simulink model "traj_model_pid"  (R2022b)
settings: Solver=VariableStepAuto  StartTime=0.0  StopTime=10.0  RelTol=1e-3
values from neighbouring files (symbols this model uses):
  L = 235    [trajectory_script.m]
  v_d = 100    [trajectory_script.m]
settings Model: Creator=hamra  LastModifiedBy=hamra

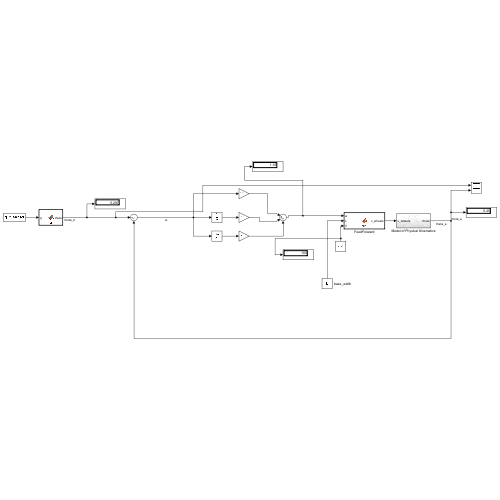
[thumbnail: Simulink's stored preview of the top-level diagram]
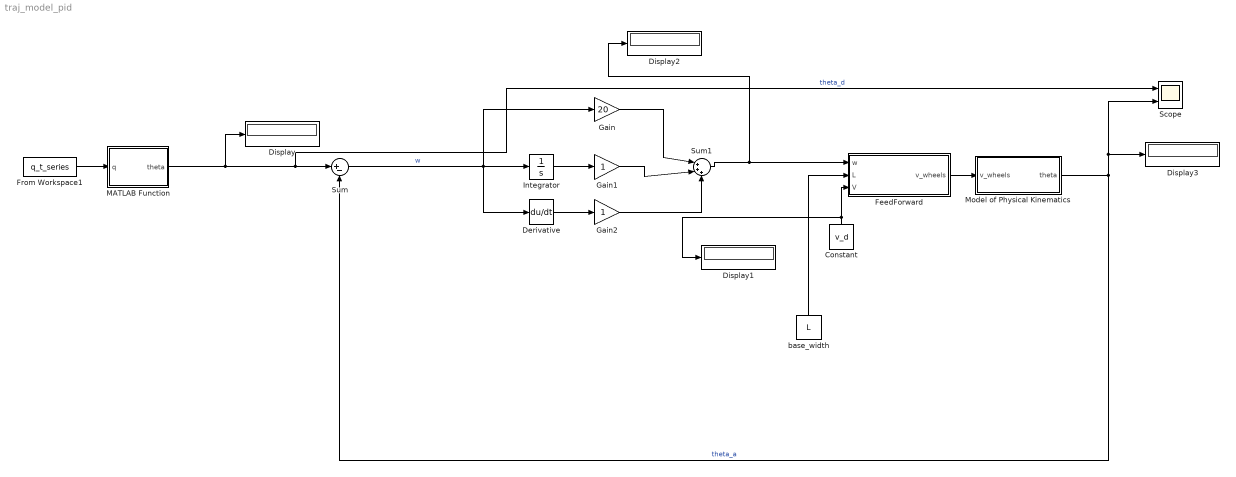
== system traj_model_pid ==
  Constant : Constant  Value=v_d
  Derivative : Derivative
  Display{,1..3} (4 alike) : Display
  FeedForward : MATLAB Function  TreatAsAtomicUnit=on
  From Workspace1 : FromWorkspace  VariableName=q_t_series
  Gain : Gain  Gain=20
  Gain1 : Gain
  Gain2 : Gain
  Integrator : Integrator
  MATLAB Function : MATLAB Function  TreatAsAtomicUnit=on
  Model of Physical Kinematics : Subsystem
  Scope : Scope  NumInputPorts=2
  Sum : Sum  Inputs=|+-
  Sum1 : Sum  Inputs=|+++
  base_width : Constant  Value=L
  wires:
  From Workspace1/1 -> MATLAB Function/1(q)
  Sum/1 -> Derivative/1, Gain/1, Integrator/1  "w"
  Derivative/1 -> Gain2/1
  Integrator/1 -> Gain1/1
  Gain/1 -> Sum1/1
  Gain1/1 -> Sum1/2
  Gain2/1 -> Sum1/3
  base_width/1 -> FeedForward/2(L)
  FeedForward/1(v_wheels) -> Model of Physical Kinematics/1(v_wheels)
  Constant/1 -> FeedForward/3(V), Display1/1
  Model of Physical Kinematics/1(theta) -> Scope/2, Display3/1, Sum/2  "theta_a"
  MATLAB Function/1(theta) -> Display/1, Scope/1, Sum/1  "theta_d"
  Sum1/1 -> Display2/1, FeedForward/1(w)

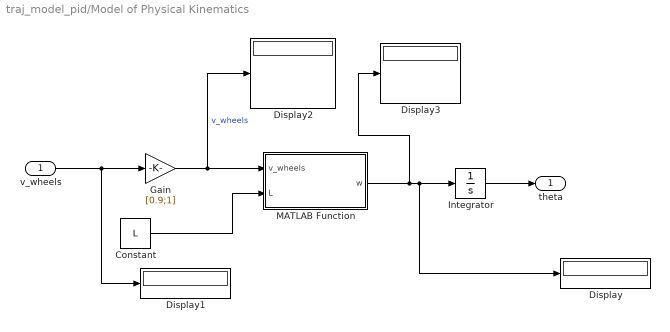
== system traj_model_pid/Model of Physical Kinematics ==
  v_wheels : Inport
  Constant : Constant  Value=L
  Display{,1..3} (4 alike) : Display
  Gain : Gain  Gain=[0.9;1]
  Integrator : Integrator
  MATLAB Function : MATLAB Function  TreatAsAtomicUnit=on
  theta : Outport
  wires:
  Constant/1 -> MATLAB Function/2(L)
  MATLAB Function/1(w) -> Display3/1, Display/1, Integrator/1
  Gain/1 -> Display2/1, MATLAB Function/1(v_wheels)  "v_wheels"
  Integrator/1 -> theta/1
  v_wheels/1 -> Display1/1, Gain/1

== matlab function traj_model_pid/MATLAB Function ==
  data: q input; theta output
function theta = fcn(q)

theta = q(3);

== matlab function traj_model_pid/Model of Physical Kinematics/MATLAB Function ==
  data: v_wheels input; w output; L input
function w = fcn(v_wheels, L)

v_r = v_wheels(1);
v_l = v_wheels(2);

w = (v_r - v_l)/L;

== matlab function traj_model_pid/FeedForward ==
  data: w input; v_wheels output; L input; V input
function v_wheels = fcn(w,L, V)
%L = 235; %nominal base width [mm]


v_1 = V + L/2*w; %right velocity [mm/s]
v_2 = V - L/2*w; %left velocity [mm/s]
v_wheels = [v_1;v_2]; %velocity vector
